simulink model "NewMain"  (R2024b)
settings: Solver=VariableStepAuto  StartTime=0.0  StopTime=5  RelTol=1e-3
libraries: robotmaniplib x5, robotcorelib x3, slpidlib x1, dspinverses x1, robotsim3dlib x1, sim3dlib x1
settings Model: Creator=jc5724  LastModifiedBy=dd217

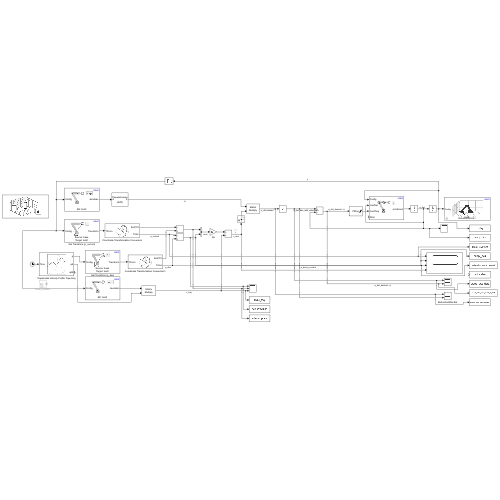
[thumbnail: Simulink's stored preview of the top-level diagram]
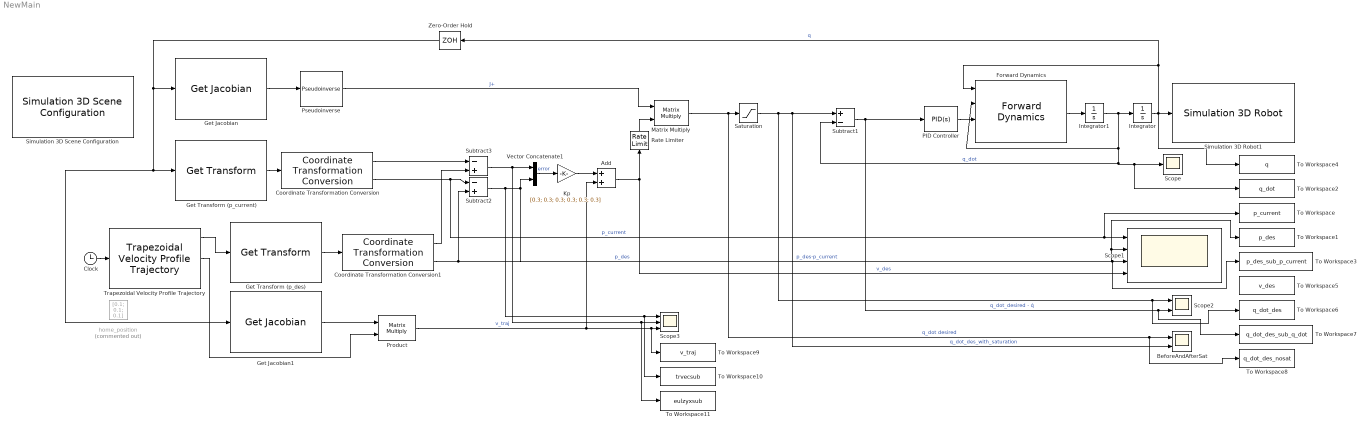
== system NewMain ==
  Add : Sum
  BeforeAndAfterSat : Scope  NumInputPorts=2
  Clock : Clock
  Coordinate Transformation Conversion : robotcorelib/Coordinate Transformation Conversion  InputRepresentation=Homogeneous Transformation  InputEulerSequence=ZYX  ShowTrVecInputPort=on  OutputRepresentation=Euler Angles  OutputEulerSequence=ZYX  ShowTrVecOutputPort=on  SimulateUsing=Interpreted execution
  Coordinate Transformation Conversion1 : robotcorelib/Coordinate Transformation Conversion  InputRepresentation=Homogeneous Transformation  InputEulerSequence=ZYX  ShowTrVecInputPort=on  OutputRepresentation=Euler Angles  OutputEulerSequence=ZYX  ShowTrVecOutputPort=on  SimulateUsing=Interpreted execution
  Forward Dynamics : robotmaniplib/Forward Dynamics  RigidBodyTree=robot  SimulateUsing=Interpreted execution
  Get Jacobian : robotmaniplib/Get Jacobian  RigidBodyTree=robot  EndEffector=tool0  SimulateUsing=Interpreted execution
  Get Jacobian1 : robotmaniplib/Get Jacobian  RigidBodyTree=robot  EndEffector=tool0  SimulateUsing=Interpreted execution
  Get Transform (p_current) : robotmaniplib/Get Transform  RigidBodyTree=robot  SourceBody=base  TargetBody=tool0  SimulateUsing=Interpreted execution
  Get Transform (p_des) : robotmaniplib/Get Transform  RigidBodyTree=robot  SourceBody=base  TargetBody=tool0  SimulateUsing=Interpreted execution
  Integrator : Integrator  InitialCondition=[0;0;0;0;0;0]
  Integrator1 : Integrator  InitialCondition=[0;0;0;0;0;0]
  Kp : Gain  Gain=[0.3; 0.3; 0.3; 0.3; 0.3; 0.3]
  Matrix Multiply : Product  Multiplication=Matrix(*)
  PID Controller : slpidlib/PID Controller  Controller=PID  Form=Parallel  TimeDomain=Continuous-time  UseExternalTs=off  SampleTime=-1  IntegratorMethod=Forward Euler  FilterMethod=Forward Euler  ControllerParametersSource=internal  P=2  I=0.3  UseKiTs=off  D=0.1  UseExternalDerivativeSource=off  N=50  UseFilter=on  TunerSelectOption=Transfer Function Based (PID Tuner App)  InitialConditionSource=internal  InitialConditionForIntegrator=0  InitialConditionForFilter=0  DifferentiatorICPrevScaledInput=0  ExternalReset=none  TrackingMode=off  Kt=1  LimitOutput=on  SatLimitsSource=internal  UpperSaturationLimit=3  LowerSaturationLimit=-3  LinearizeAsGain=on  AntiWindupMode=back-calculation  Kb=1  LimitIntegrator=off  UpperIntegratorSaturationLimit=inf  LowerIntegratorSaturationLimit=-inf  POutMin=[]  POutMax=[]  IOutMin=[]  IOutMax=[]  DOutMin=[]  DOutMax=[]  NOutMin=[]  NOutMax=[]  SumOutMin=[]  SumOutMax=[]  SaturationOutMin=[]  SaturationOutMax=[]  PParamMin=[]  PParamMax=[]  IParamMin=[]  IParamMax=[]  DParamMin=[]  DParamMax=[]  NParamMin=[]  NParamMax=[]  KbParamMin=[]  KbParamMax=[]  KtParamMin=[]  KtParamMax=[]  KbOutMin=[]  KbOutMax=[]  KtOutMin=[]  KtOutMax=[]  IntegratorOutMin=[]  IntegratorOutMax=[]  FilterOutMin=[]  FilterOutMax=[]  SumI1OutMin=[]  SumI1OutMax=[]  SumI2OutMin=[]  SumI2OutMax=[]  SumI3OutMin=[]  SumI3OutMax=[]  SumI4OutMin=[]  SumI4OutMax=[]  SumDOutMin=[]  SumDOutMax=[]  DifferentiatorOutMin=[]  DifferentiatorOutMax=[]  FilterDiffOutCoefMin=[]  FilterDiffOutCoefMax=[]  ReciprocalOutMin=[]  ReciprocalOutMax=[]  SumDenOutMin=[]  SumDenOutMax=[]  SumNumOutMin=[]  SumNumOutMax=[]  DivideOutMin=[]  DivideOutMax=[]  UdiffTsProdOutMin=[]  UdiffTsProdOutMax=[]  NTsProdOutMin=[]  NTsProdOutMax=[]  UintegralTsProdOutMin=[]  UintegralTsProdOutMax=[]  UngainTsProdOutMin=[]  UngainTsProdOutMax=[]  ClampingZeroOutDataTypeStr=Inherit: Inherit via back propagation  ClampingZeroOutMin=[]  ClampingZeroOutMax=[]  FilterDenConstantOutDataTypeStr=Inherit: Inherit via back propagation  FilterDenConstantOutMin=[]  FilterDenConstantOutMax=[]  PCopyOutDataTypeStr=Inherit: Inherit via back propagation  PCopyOutMin=[]  PCopyOutMax=[]  NCopyOutDataTypeStr=Inherit: Inherit via back propagation  NCopyOutMin=[]  NCopyOutMax=[]  IntegratorContinuousStateAttributes=''  IntegratorStateMustResolveToSignalObject=off  IntegratorRTWStateStorageClass=Auto  FilterContinuousStateAttributes=''  FilterStateMustResolveToSignalObject=off  FilterRTWStateStorageClass=Auto  ParallelPVariant=InternalParameters  IdealPVariant=Disabled  IVariant=InternalParameters  DVariant=InternalParameters  IntegratorVariant=Continuous  SatVariant=Enabled  AWVariant=BackCalculation  PCopyVariant=Disabled  TRVariant=Disabled  FdbkBlocksVariant=Forward  IdealPFdbkVariant=Disabled  SatFdbkVariant=Disabled  DerivativeFilterVariant=ContFilter  NVariant=InternalParameters  NCopyVariant=Disabled  FilterICVariant=InternalICsFilter  IntegratorICVariant=InternalICs  ExternalResetVariant=Disabled  TRSumVariant=Passthrough  SumFdbkVariant=Disabled  SumVariant=Sum_PID  TsampFilterVariant=InternalTs  TsampNgainVariant=Passthrough  TsampIntegralVariant=Disabled_SignalSpec  ExternalSaturationOutDataTypeStr=Inherit: Same as second input  DerivativeSourceVariant=ErrorSignal  PreIntVariant=InternalPreInt
  Product : Product  Multiplication=Matrix(*)
  Pseudoinverse : dspinverses/Pseudoinverse  wanterr=off  SimulateUsing=Interpreted execution
  Rate Limiter : RateLimiter  RisingSlewLimit=2  FallingSlewLimit=-2  SampleTimeMode=inherited
  Saturation : Saturate  UpperLimit=3  LowerLimit=-3
  Scope : Scope
  Scope1 : Scope  NumInputPorts=4
  Scope2 : Scope  NumInputPorts=2
  Scope3 : Scope  NumInputPorts=3
  Simulation 3D Robot1 : robotsim3dlib/Simulation 3D Robot  actorInputType=RigidBodyTree Object  RigidBodyTree=robot  ActorName=SimulinkVehicle1  existActorChekBox=off  initialTrans=[0 0 0]  initialRot=[0 0 0]  initialConfig="[0  0  0  0  0  0]"  EndEffector=tool0  eeOffsetInpChekBox=off  eeTargetTrans=[0 0 0]  eeTargetRot=[0 0 0]  enableRegionGraspChekBox=off  regionGraspInpChekBox=off  eeTargTransDiff=[0.2 0.2 0.2]  eeTargRotDiff=[0 0 0]  inpConfEnbVal=on  inpGraspEnbVal=off  inpTransEnbVal=off  outConfEnbVal=off  outGraspEnbVal=off  outTransEnbVal=off  SampleTime=0.01  ActorType=SimulinkVehicle  ID=1  aMode=6  ActorTag=SimulinkVehicle1  Mesh=RigidBodyTree
  Simulation 3D Scene Configuration : sim3dlib/Simulation 3D Scene Configuration  Priority=-1  ProjectFormat=Default Scenes  SceneDesc=Empty scene  ProjectName=C:\Program Files\MATLAB\R2024b\toolbox\shared\sim3d_projects\automotive_project_windows\UE\WindowsNoEditor\VehicleSimulation.exe  ScenePath=/Game/Maps/EmptyScene  EnableOpenDRIVE=off  vehTagList={'<empty>';'Scene Origin';'SimulinkVehicle1'}  vehTag=Scene Origin  FreeCameraInitialTranslation=[0, 0, 0]  FreeCameraDefaultInitialTranslation=[-6, 0, 2]  FreeCameraInitialRotation=[0, 0, 0]  FreeCameraDefaultInitialRotation=[0, -15, 0]  OpVisEn=off  Ts=0.01  EnableWindow=on  EnableRemoteAccess=off  EnableWeather=off  SunAzimuth=90  SunAltitude=40.0  EnableGeospatialSun=off  Latitude=0  Longitude=0  Date=2023-01-01  Time=10:30:00  GeoTimeZone=-5.0  SunDaylightSaving=off  wind=1  clouds=10  EnableVolumetricClouds=off  CloudCoverage=0  CloudAltitude=6  fog=0  rain=0  RaindropsEffect=off  SnowDensity=0  EnableGeospatial=off  UseTrueOrigin=off  OriginHeight=200  OriginLatitude=40.744652  OriginLongitude=-73.988864  MapStyle=Aerial  AdditionalAssetIDs=[]  UseAdvancedSunSky=off  SolarTime=11  TimeZone=-5  Day=21  Month=9  Year=2022  UseDaylightSavingTime=on  DSTStartDay=10  DSTStartMonth=3  DSTEndDay=3  DSTEndMonth=11  DSTSwitchHour=2  sensorTag=MainCamera1  sensorId=1  sensorName=MainCamera1  mountLoc=Origin  offsetFlag=off  tmountOffset=[0, 0, 0]  rmountOffset=[0, 0, 0]  HorizontalResolution=1280  VerticalResolution=720  HorizontalFOV=60  mountPoint=[0 0 0]  mountOrientation=[0 0 0]  aMode=6  ID=1  GeoTrigger=Inactive
      settings: LibrarySourceBlock=robotsim3dlib/Simulation 3D Scene Configuration
  Subtract1 : Sum  Inputs=+-
  Subtract2 : Sum  Inputs=-+
  Subtract3 : Sum  Inputs=-+
  To Workspace : ToWorkspace  VariableName=p_current  SaveFormat=Structure With Time  SampleTime=0.01
  To Workspace1 : ToWorkspace  VariableName=p_des  SaveFormat=Structure With Time  SampleTime=0.01
  To Workspace10 : ToWorkspace  VariableName=trvecsub  SaveFormat=Structure With Time  SampleTime=0.01
  To Workspace11 : ToWorkspace  VariableName=eulzyxsub  SaveFormat=Structure With Time  SampleTime=0.01
  To Workspace2 : ToWorkspace  VariableName=q_dot  SaveFormat=Structure With Time  SampleTime=0.01
  To Workspace3 : ToWorkspace  VariableName=p_des_sub_p_current  SaveFormat=Structure With Time  SampleTime=0.01
  To Workspace4 : ToWorkspace  VariableName=q  SaveFormat=Structure With Time  SampleTime=0.01
  To Workspace5 : ToWorkspace  VariableName=v_des  SaveFormat=Structure With Time  SampleTime=0.01
  To Workspace6 : ToWorkspace  VariableName=q_dot_des  SaveFormat=Structure With Time  SampleTime=0.01
  To Workspace7 : ToWorkspace  VariableName=q_dot_des_sub_q_dot  SaveFormat=Structure With Time  SampleTime=0.01
  To Workspace8 : ToWorkspace  VariableName=q_dot_des_nosat  SaveFormat=Structure With Time  SampleTime=0.01
  To Workspace9 : ToWorkspace  VariableName=v_traj  SaveFormat=Structure With Time  SampleTime=0.01
  Trapezoidal Velocity Profile Trajectory : robotcorelib/Trapezoidal Velocity Profile Trajectory  WaypointSource=Internal  Waypoints=|  NumParams=2  Parameter1=Peak Velocity  Parameter2=Acceleration  ParameterSource=Internal  PeakVelocity=[0.02; 0.02; 0.02; 0.02; 0.02; 0.02]  Acceleration=[0.1; 0.1; 0.1; 0.1; 0.1; 0.1]  EndTime=[ 1; 1 ]  AccelTime=[ 1; 2 ]  SimulateUsing=Interpreted execution
      | [0 0.2 0.4 0.6;
      |  0 -0.2 -0.4 -0.6;
      |  0 0.1 0.2 0.3;
      |  0 -0.1 -0.2 -0.3;
      |  0 0 0 0;
      |  0 0 0 0]
  Vector Concatenate1 : Concatenate
  Zero-Order Hold : ZeroOrderHold  SampleTime=-1
  home_position : Constant  Commented=on  Value=[0.1; 0.1; 0.1]
  wires:
  Zero-Order Hold/1 -> Get Jacobian/1, Get Jacobian1/1, Get Transform (p_current)/1
  Clock/1 -> Trapezoidal Velocity Profile Trajectory/1
  PID Controller/1 -> Forward Dynamics/3
  Subtract1/1 -> To Workspace7/1, Scope2/2, PID Controller/1  "q_dot_desired - q̇"
  Integrator1/1 -> To Workspace2/1, Scope/1, Subtract1/2, Forward Dynamics/2, Integrator/1  "q_dot"
  Pseudoinverse/1 -> Matrix Multiply/1  "J+"
  Get Jacobian/1 -> Pseudoinverse/1
  Matrix Multiply/1 -> Saturation/1, To Workspace8/1, BeforeAndAfterSat/1  "q_dot desired"
  Saturation/1 -> Subtract1/1, BeforeAndAfterSat/2, To Workspace6/1, Scope2/1  "q_dot_des_with_saturation"
  Rate Limiter/1 -> Matrix Multiply/2
  Coordinate Transformation Conversion/2 -> To Workspace/1, Scope1/1, Subtract2/1  "p_current"
  Get Transform (p_current)/1 -> Coordinate Transformation Conversion/1
  Coordinate Transformation Conversion1/2 -> Subtract2/2, To Workspace1/1, Scope1/2  "p_des"
  Integrator/1 -> Zero-Order Hold/1, Forward Dynamics/1, To Workspace4/1, Simulation 3D Robot1/1  "q"
  Get Transform (p_des)/1 -> Coordinate Transformation Conversion1/1
  Forward Dynamics/1 -> Integrator1/1
  Subtract2/1 -> To Workspace10/1, Scope3/1, Vector Concatenate1/2, To Workspace3/1, Scope1/3  "p_des-p_current"
  Coordinate Transformation Conversion/1 -> Subtract3/1
  Coordinate Transformation Conversion1/1 -> Subtract3/2
  Trapezoidal Velocity Profile Trajectory/1 -> Get Transform (p_des)/1
  Get Jacobian1/1 -> Product/1
  Trapezoidal Velocity Profile Trajectory/2 -> Product/2
  Subtract3/1 -> To Workspace11/1, Scope3/2, Vector Concatenate1/1
  Vector Concatenate1/1 -> Kp/1  "error"
  Product/1 -> Add/2, To Workspace9/1, Scope3/3  "v_traj"
  Kp/1 -> Add/1
  Add/1 -> Scope1/4, Rate Limiter/1  "v_des"
